simulink model "problem3"  (R2020b)
settings: Solver=VariableStepAuto  StartTime=0.0  StopTime=10.0  RelTol=1e-3
PreLoadFcn:
  | % Load initialization data
  | 
  | problem3;
values from neighbouring files (symbols this model uses):
  ctrl = 0    [ABS_code.m]    (also in abs_datadictionary.sldd = 1.0; init_data.m = 1)
  g = 32.18    [abs_datadictionary.sldd]    (also in init_data.m)
  Kf = 1.0    [abs_datadictionary.sldd]    (also in init_data.m = 1)
  l = 5.0    [abs_datadictionary.sldd]
  m = 50.0    [abs_datadictionary.sldd]    (also in init_data.m = 50)
  mu = 0.0 0.4 0.8 0.97 1.0 0.98 0.96 0.94 0.92 0.9 0.88 0.855 0.83 0.81 0.79 0.77 0.75 0.73 0.72 0.71 0.7    [abs_datadictionary.sldd]    (also in init_data.m = [0 .4 .8 .97 1.0 .98 .96 .94 .92 .9 .88 .855 .83 .81 .79 .77)
  PBmax = 1500.0    [abs_datadictionary.sldd]    (also in init_data.m = 1500)
  Rr = 1.25    [abs_datadictionary.sldd]    (also in init_data.m)
  slip = 0.0 0.05 0.1 0.15000000000000002 0.2 0.25 0.30000000000000004 0.35000000000000003 0.4 0.45 0.5 0.55 0.6 0.64999999999999991 0.7 0.75 0.8 0.85 0.9 0.95 1.0    [abs_datadictionary.sldd]    (also in init_data.m = (0:.05:1.0))
  TB = 0.01    [abs_datadictionary.sldd]    (also in init_data.m)
  v0 = 88.0    [abs_datadictionary.sldd]    (also in init_data.m = 88)
settings Model: DataDictionary=abs_datadictionary.sldd  Creator=Sourav Kumar  LastModifiedBy=Sourav Kumar

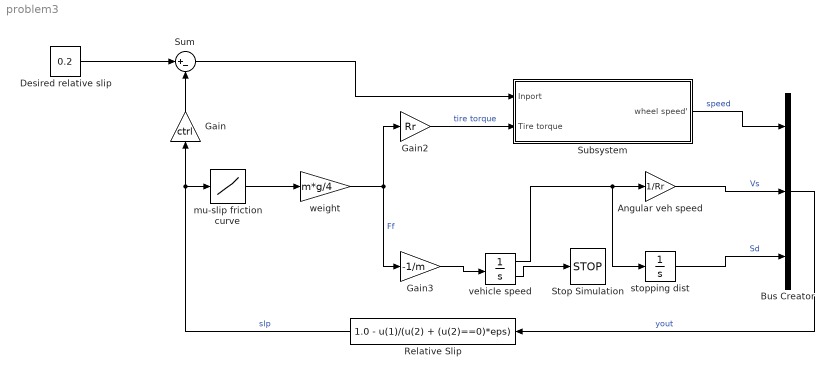
== system problem3 ==
  Angular veh speed : Gain  Gain=1/Rr
  Bus Creator : BusCreator  Inputs=3
  Desired relative slip : Constant  Value=0.2
  Gain : Gain  Gain=ctrl
  Gain2 : Gain  Gain=Rr
  Gain3 : Gain  Gain=-1/m
  Relative Slip : Fcn  Expr=1.0 - u(1)/(u(2) + (u(2)==0)*eps)
  Stop Simulation : Stop
  Subsystem : Subsystem
  Sum : Sum  Inputs=|+-
  "mu-slip friction curve " : Lookup_n-D  NumberOfTableDimensions=1  BreakpointsForDimension1=slip  Table=mu  InternalRulePriority=Speed  RndMeth=Simplest  InputSameDT=on
  stopping dist : Integrator
  vehicle speed : Integrator  InitialCondition=v0  LimitOutput=on  UpperSaturationLimit=1000  LowerSaturationLimit=0  ShowSaturationPort=on
  weight : Gain  Gain=m*g/4
  wires:
  vehicle speed/1 -> stopping dist/1, Angular veh speed/1
  Desired relative slip/1 -> Sum/1
  Gain/1 -> Sum/2
  Relative Slip/1 -> "mu-slip friction curve "/1, Gain/1  "slp"
  "mu-slip friction curve "/1 -> weight/1
  weight/1 -> Gain3/1, Gain2/1  "Ff"
  Gain3/1 -> vehicle speed/1
  Angular veh speed/1 -> Bus Creator/2  "Vs"
  stopping dist/1 -> Bus Creator/3  "Sd"
  Bus Creator/1 -> Relative Slip/1  "yout"
  Gain2/1 -> Subsystem/2(Tire torque)  "tire torque"
  Sum/1 -> Subsystem/1(Inport)
  Subsystem/1(wheel speed') -> Bus Creator/1  "speed"
  vehicle speed/2 -> Stop Simulation/1

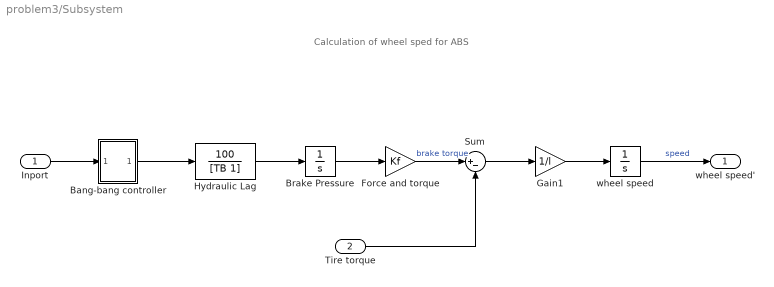
== system problem3/Subsystem ==
  note: Calculation of wheel sped for ABS
  Inport : Inport
  Tire torque : Inport  Port=2
  Bang-bang controller : Subsystem  mask(Sign){}
      mask help: y = sign(x)
      mask Help: Sign Function:\n\t\t\ty = 1 if x > 0\n\t\t\ty = 0 if x = 0\n\t\t\ty = -1 if x < 0
      mask Display: plot(-50,-50,50,50,[-50,50],[0,0],[0,0],[-50,50],[-40,0],[-30,-30],[0,40],[30,30])
  Brake Pressure : Integrator  LimitOutput=on  UpperSaturationLimit=PBmax  LowerSaturationLimit=0
  Force and torque : Gain  Gain=Kf
  Gain1 : Gain  Gain=1/l
  Hydraulic Lag : TransferFcn  Numerator=[100]  Denominator=[TB 1]
  Sum : Sum  Inputs=|+-
  wheel speed : Integrator  InitialCondition=v0/Rr  LimitOutput=on  UpperSaturationLimit=1000  LowerSaturationLimit=0
  wheel speed' : Outport
  wires:
  Brake Pressure/1 -> Force and torque/1
  Sum/1 -> Gain1/1
  Bang-bang controller/1(out_1) -> Hydraulic Lag/1
  wheel speed/1 -> wheel speed'/1  "speed"
  Tire torque/1 -> Sum/2
  Gain1/1 -> wheel speed/1
  Inport/1 -> Bang-bang controller/1(in_1)
  Hydraulic Lag/1 -> Brake Pressure/1
  Force and torque/1 -> Sum/1  "brake torque"

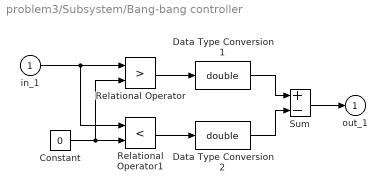
== system problem3/Subsystem/Bang-bang controller ==
  in_1 : Inport
  Constant : Constant  Value=0
  Data Type Conversion1 : DataTypeConversion  OutDataTypeStr=double  SaturateOnIntegerOverflow=on  RndMeth=Zero
  Data Type Conversion2 : DataTypeConversion  OutDataTypeStr=double  SaturateOnIntegerOverflow=on  RndMeth=Zero
  Relational Operator : RelationalOperator  Operator=>  OutDataTypeStr=boolean  RndMeth=Nearest  InputSameDT=on
  Relational Operator1 : RelationalOperator  Operator=<  OutDataTypeStr=boolean  RndMeth=Nearest  InputSameDT=on
  Sum : Sum  Inputs=+-  InputSameDT=on  SaturateOnIntegerOverflow=on  OutDataTypeStr=Inherit: Same as first input
  out_1 : Outport  InitialOutput=0  VectorParamsAs1DForOutWhenUnconnected=off
  wires:
  Data Type Conversion2/1 -> Sum/2
  Data Type Conversion1/1 -> Sum/1
  Sum/1 -> out_1/1
  Relational Operator/1 -> Data Type Conversion1/1
  Relational Operator1/1 -> Data Type Conversion2/1
  Constant/1 -> Relational Operator/2, Relational Operator1/2
  in_1/1 -> Relational Operator1/1, Relational Operator/1
